simulink model "rigidBodyControl"  (R2016b)
settings: Solver=VariableStepAuto  StartTime=0.0  StopTime=0.1  FixedStep=2e-4  MaxStep=1e-6  RelTol=1e-3
values from neighbouring files (symbols this model uses):
  denGc = denGc{1}    [rigidBodyInit.m]
  denGp = [m0 0 0]    [rigidBodyInit.m]
  numGc = numGc{1}    [rigidBodyInit.m]
  numGp = [1]    [rigidBodyInit.m]
  TsN = 1e-6    (= 1e-06)    [rigidBodyInit.m]
libraries: model_controller x2, simulink x1
settings Model: Creator=Dai Luyao  LastModifiedBy=Dai Luyao

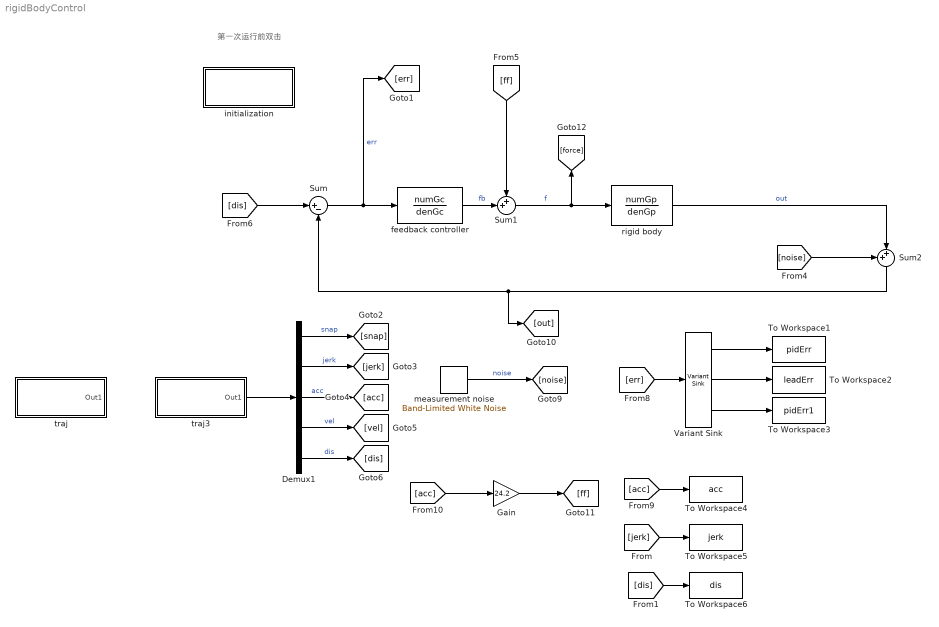
== system rigidBodyControl ==
  note: 第一次运行前双击
  Demux1 : Demux  Outputs=5
  Gain : Gain  Gain=24.2
  Sum : Sum  Inputs=|+-
  Sum1 : Sum  Inputs=++|
  Sum2 : Sum  Inputs=++|
  To Workspace1 : ToWorkspace  VariableName=pidErr  SaveFormat=Structure With Time  SampleTime=-1
  To Workspace2 : ToWorkspace  VariableName=leadErr  SaveFormat=Structure With Time  SampleTime=-1
  To Workspace3 : ToWorkspace  VariableName=pidErr1  SaveFormat=Structure With Time  SampleTime=-1
  To Workspace4 : ToWorkspace  VariableName=acc  SaveFormat=Structure With Time  SampleTime=-1
  To Workspace5 : ToWorkspace  VariableName=jerk  SaveFormat=Structure With Time  SampleTime=-1
  To Workspace6 : ToWorkspace  VariableName=dis  SaveFormat=Structure With Time  SampleTime=-1
  Variant Sink : VariantSink
  feedback controller : TransferFcn  Numerator=numGc  Denominator=denGc
  initialization : Subsystem
      settings: OpenFcn=rigidBodyInit;  MoveFcn=edit rigidBodyInit;
  measurement noise : simulink/Sources/Band-Limited White Noise  Cov=noisePower  Ts=TsN  seed=[23341]
  rigid body : TransferFcn  Numerator=numGp  Denominator=denGp
  traj : Subsystem  BlockChoice=4th order traj
      link override 3rd order traj: j=800  v=0.25  x=0.06  a=10
      settings: AttributesFormatString=%<BlockChoice>  TemplateBlock=model_controller/Profile Generators/traj  MemberBlocks=2th order traj,3rd order traj,4th order traj,step
  traj3 : Subsystem  BlockChoice=4th order traj
      link override 4th order traj: v=0.25  x=0.001  a=20  d=200000  j=1200
      settings: AttributesFormatString=%<BlockChoice>  TemplateBlock=model_controller/Profile Generators/traj  MemberBlocks=2th order traj,3rd order traj,4th order traj,step
  wires:
  Sum/1 -> feedback controller/1, [err]  "err"
  feedback controller/1 -> Sum1/2  "fb"
  Sum1/1 -> rigid body/1, [force]  "f"
  [dis] -> Sum/1
  measurement noise/1 -> [noise]  "noise"
  rigid body/1 -> Sum2/2  "out"
  Sum2/1 -> [out], Sum/2
  Demux1/1 -> [snap]  "snap"
  Demux1/2 -> [jerk]  "jerk"
  Demux1/3 -> [acc]  "acc"
  Demux1/4 -> [vel]  "vel"
  Demux1/5 -> [dis]  "dis"
  [err] -> Variant Sink/1
  Variant Sink/1 -> To Workspace1/1
  Variant Sink/2 -> To Workspace2/1
  Variant Sink/3 -> To Workspace3/1
  [acc] -> To Workspace4/1
  Gain/1 -> [ff]
  [acc] -> Gain/1
  [jerk] -> To Workspace5/1
  traj3/1(Out1) -> Demux1/1
  [ff] -> Sum1/1
  [noise] -> Sum2/1
  [dis] -> To Workspace6/1

== system rigidBodyControl/initialization ==

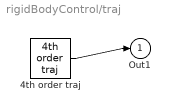
== system rigidBodyControl/traj ==
  4th order traj : model_controller/Profile Generators/4th order traj  t0=0  x=0.06  v=0.25  a=10  j=800  d=64000  Ts=0
  Out1 : Outport
  wires:
  4th order traj/1 -> Out1/1

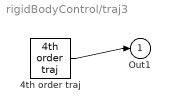
== system rigidBodyControl/traj3 ==
  4th order traj : model_controller/Profile Generators/4th order traj  t0=0  x=0.001  v=0.25  a=20  j=1200  d=200000  Ts=0
  Out1 : Outport
  wires:
  4th order traj/1 -> Out1/1
